simulink model "emt_short_transm_line"  (R2019a)
settings: Solver=VariableStepAuto  StartTime=0.0  StopTime=1.0  RelTol=1e-3
libraries: powerlib x7, powerlib_meascontrol x6
settings Model: Creator=Psyna  LastModifiedBy=Psyna

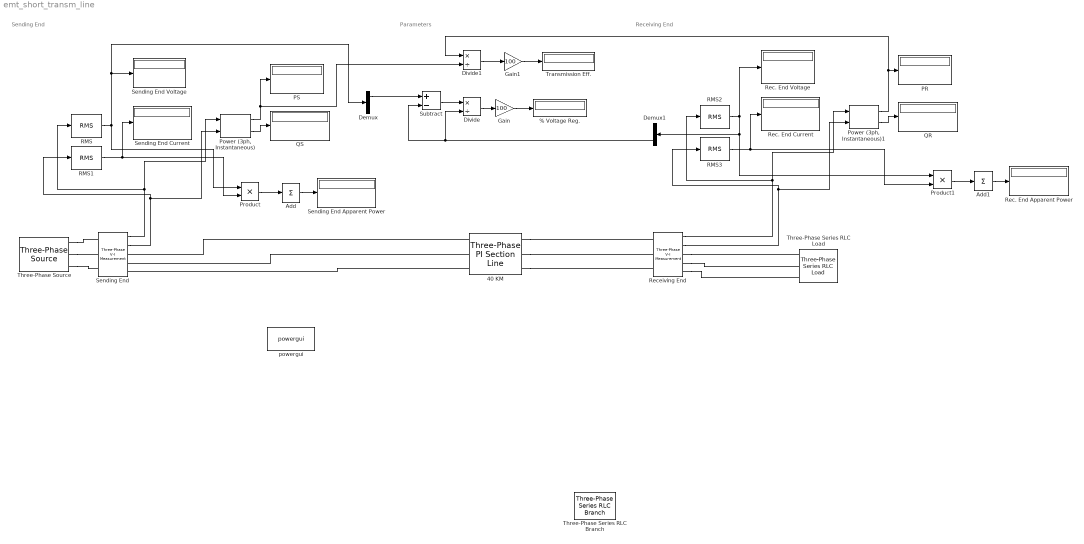
== system emt_short_transm_line ==
  note: Parameters
  note: Receiving End
  note: Sending End
  % Voltage Reg. : Display
  40 KM : powerlib/Elements/Three-Phase PI Section Line  LConnTagsString=a|b|c  RConnTagsString=A|B|C  Frequency=60  Resistances=[ 0.15 0]  Inductances="[ 1.3263e-3  0.1]"  Capacitances=[12.74e-9 7.751e-9]  Length=40
      settings: SourceProductName=Simscape Electrical
  Add : Sum  Inputs=+
  Add1 : Sum  Inputs=+
  Demux : Demux  Outputs=3
  Demux1 : Demux  Outputs=3
  Divide : Product  Inputs=*/
  Divide1 : Product  Inputs=*/
  Gain : Gain  Gain=100
  Gain1 : Gain  Gain=100
  PR : Display
  PS : Display
  "Power (3ph, Instantaneous)" : powerlib_meascontrol/Measurements/Power (3ph, Instantaneous)
      settings: SourceProductName=Simscape Electrical
  "Power (3ph, Instantaneous)1" : powerlib_meascontrol/Measurements/Power (3ph, Instantaneous)
      settings: SourceProductName=Simscape Electrical
  Product : Product
  Product1 : Product
  QR : Display
  QS : Display
  RMS{,1..3} (4 alike) : powerlib_meascontrol/Measurements/RMS  TrueRMS=on  Freq=60  RMSInit=0  Ts=0
      settings: SourceProductName=Simscape Electrical
  Rec. End Apparent Power : Display
  Rec. End Current : Display
  Rec. End Voltage : Display
  Receiving End : powerlib/Measurements/Three-Phase V-I Measurement  VoltageMeasurement=phase-to-ground  SetLabelV=off  LabelV=Vabc  Vpu=off  VpuLL=off  CurrentMeasurement=yes  SetLabelI=off  LabelI=Iabc  Ipu=off  Pbase=100e6  Vbase=500e3  OutputType=Complex  PhasorSimulation=off  PSBequivalent=0
      settings: SourceProductName=Simscape Electrical
  "Sending End " : powerlib/Measurements/Three-Phase V-I Measurement  VoltageMeasurement=phase-to-ground  SetLabelV=off  LabelV=Vabc  Vpu=off  VpuLL=off  CurrentMeasurement=yes  SetLabelI=off  LabelI=Iabc  Ipu=off  Pbase=100e6  Vbase=500e3  OutputType=Complex  PhasorSimulation=off  PSBequivalent=0
      settings: SourceProductName=Simscape Electrical
  Sending End Apparent Power : Display
  Sending End Current : Display
  Sending End Voltage : Display
  Subtract : Sum  Inputs=+-
  Three-Phase Series RLC Branch : powerlib/Elements/Three-Phase Series RLC Branch  LConnTagsString=A|B|C  RConnTagsString=A|B|C  BranchType=RL  Resistance=6  Inductance=0.053052  Capacitance=1e-6  Measurements=None
      settings: SourceProductName=Simscape Electrical
  Three-Phase Series RLC Load : powerlib/Elements/Three-Phase Series RLC Load  LConnTagsString=A|B|C  Configuration=Y (grounded)  NominalVoltage=220e3  Vabc=[1e3 1e3 1e3]  Vabcp=[1e3 1e3 1e3]  NominalFrequency=60  UnbalancedPower=off  ActivePower=304.8e6  InductivePower=228.6e6  CapacitivePower=0  Pabc=[10e3 9e3 11e3]  QLabc=[100 90 110]  QCabc=[100 90 110]  Pabcp=[10e3 9e3 11e3]  QLabcp=[100 90 110]  QCabcp=[100 90 110]  Measurements=None  LoadType=constant Z
      settings: SourceProductName=Simscape Electrical
  Three-Phase Source : powerlib/Electrical Sources/Three-Phase Source  InternalConnection=Yg  VoltagePhases=off  Voltage=250e3  PhaseAngle=0  Voltage_phases=[25e3 25e3 25e3]/sqrt(3)  PhaseAngles_phases=[0 -120 +120]  Frequency=60  NonIdealSource=on  SpecifyImpedance=off  Resistance=0.8929  Inductance=16.58e-3  ShortCircuitLevel=100e6  BaseVoltage=25e3  XRratio=7  BusType=swing  Pref=10e3  Qref=0  Prefabc=[10e3, 10e3, 10e3]  Qrefabc=[0, 0, 0]  Qmin=-inf  Qmax=inf
      settings: SourceProductName=Simscape Electrical
  Transmission Eff. : Display
  powergui : powerlib/powergui  Priority=1  SimulationMode=Continuous  SampleTime=50e-6  frequency=60  Iterations=50  frequencyindice=60  Pbase=100e6  ErrMax=1e-4  UnitsV=kV  UnitsW=MW  buscounter=0  FunctionMessages=off  echomessages=off  EnableUseOfTLC=off  CurrentSourceSwitches=off  DisableSnubberDevices=off  DisableRonSwitches=off  DisableVfSwitches=off  DisplayEquations=off  AutomaticDiscreteSolvers=off  SolverType=Tustin/Backward Euler (TBE)  Interpol=off  ExternalGateDelay=off  methode=off  Ts=100  x0status=blocks  SPID=on  SwTol=0  HookPort=off  NonlinearTolerance=0  nMaxIteration=15  ContinueOnMaxIteration=off  RestoreLinks=warning  ResistiveCurrentMeasurement=off  Frange=[0:2:500]  Ylog=off  Xlog=on  ShowGrid=off  save=off  variable=ZData  structure=0  ZoomFFT=off  StartTime=0.0  cycles=1  DisplayStyle=1  fundamental=60  FreqAxis=off  MaxFrequency=1000  frequencyindicesteady=1  RmsSteady=1  display=off
      settings: SourceProductName=Simscape Electrical
  wires:
  "Sending End "/1 -> "Power (3ph, Instantaneous)"/1, RMS/1
  RMS/1 -> Product/1, Demux/1, Sending End Voltage/1
  RMS1/1 -> Product/2, Sending End Current/1
  "Sending End "/2 -> "Power (3ph, Instantaneous)"/2, RMS1/1
  "Power (3ph, Instantaneous)"/1 -> Divide1/2, PS/1
  "Power (3ph, Instantaneous)"/2 -> QS/1
  Product/1 -> Add/1
  Add/1 -> Sending End Apparent Power/1
  Add1/1 -> Rec. End Apparent Power/1
  Product1/1 -> Add1/1
  Receiving End/2 -> "Power (3ph, Instantaneous)1"/2, RMS3/1
  RMS3/1 -> Product1/2, Rec. End Current/1
  RMS2/1 -> Demux1/1, Product1/1, Rec. End Voltage/1
  Receiving End/1 -> "Power (3ph, Instantaneous)1"/1, RMS2/1
  "Power (3ph, Instantaneous)1"/2 -> QR/1
  "Power (3ph, Instantaneous)1"/1 -> Divide1/1, PR/1
  Demux/1 -> Subtract/1
  Demux1/3 -> Divide/2, Subtract/2
  Subtract/1 -> Divide/1
  Divide/1 -> Gain/1
  Gain/1 -> % Voltage Reg./1
  Gain1/1 -> Transmission Eff./1
  Divide1/1 -> Gain1/1
  connections:
  Three-Phase Source/RConn1 -- "Sending End "/LConn1
  Three-Phase Source/RConn3 -- "Sending End "/LConn3
  Three-Phase Source/RConn2 -- "Sending End "/LConn2
  40 KM/LConn1 -- "Sending End "/RConn1
  40 KM/LConn2 -- "Sending End "/RConn2
  40 KM/LConn3 -- "Sending End "/RConn3
  40 KM/RConn3 -- Receiving End/LConn3
  40 KM/RConn2 -- Receiving End/LConn2
  40 KM/RConn1 -- Receiving End/LConn1
  Receiving End/RConn1 -- Three-Phase Series RLC Load/LConn1
  Receiving End/RConn2 -- Three-Phase Series RLC Load/LConn2
  Receiving End/RConn3 -- Three-Phase Series RLC Load/LConn3
